simulink library "ros2lib"  (R2025a)
settings: Solver=ode45  StartTime=0.0  StopTime=10.0  RelTol=1e-3  EnableMultiTasking=on
undefined symbols (not defined in the file): coder, count, data, data_SL_Info, datatype, encoding, encoding_SL_Info, fields, fields_SL_Info, header, height, name, name_SL_Info, offset, point_step, ros, row_step, width
libraries: $bdroot x3
(part 1 of 2)
settings Model: Creator=The MathWorks, Inc.  LastModifiedBy=The MathWorks, Inc.
settings SolverCC: AlgebraicLoopSolver=TrustRegion  MaxZcPerStep=1.0
settings DataIOCC: LimitDataPoints=on  SaveFormat=Array  ReturnWorkspaceOutputs=off
settings OptimizationCC: ReuseModelBlockBuffer=off  LifeSpan=inf
settings DebuggingCC: SolverPrmCheckMsg=warning  UnconnectedInputMsg=warning  UnconnectedOutputMsg=warning  UnconnectedLineMsg=warning  AllowSymbolicDim=off  PregeneratedLibrarySubsystemCodeDiagnostic=none  SubsystemReferenceDiagnosticForUnitTest=warning  SFUnexpectedBacktrackingDiag=warning  SFNoUnconditionalDefaultTransitionDiag=warning  SFExecutionAtInitializationDiag=none  ArithmeticOperatorsInVariantConditions=warning
settings HardwareCC: ProdBitPerPointer=32.0  ProdBitPerSizeT=32.0  ProdBitPerPtrDiffT=32.0  ProdLargestAtomicFloat=None  ProdIntDivRoundTo=Undefined  ProdEndianess=Unspecified  ProdWordSize=32.0  ProdHWDeviceType=32-bit Generic
settings ModelReferenceCC: EnableRefExpFcnMdlSchedulingChecks=on  PropagateSignalLabelsOutOfModel=off
settings SFSimCC: SimUseLocalCustomCode=off
settings RTWCC: RTWUseLocalCustomCode=off  GPUComputeCapability=3.5  DLArmComputeVersion=19.05
settings CodeAppCC: StateflowObjectComments=on
settings GRTTargetCC: TargetLangStandard=C89/C90 (ANSI)
settings ConfigComp: CovScope=ReferencedModels  CovMetricSettings=dw  CovSaveCumulativeToWorkspaceVar=on  CovSaveSingleToWorkspaceVar=on  CovExternalEMLEnable=off  CovSFcnEnable=off

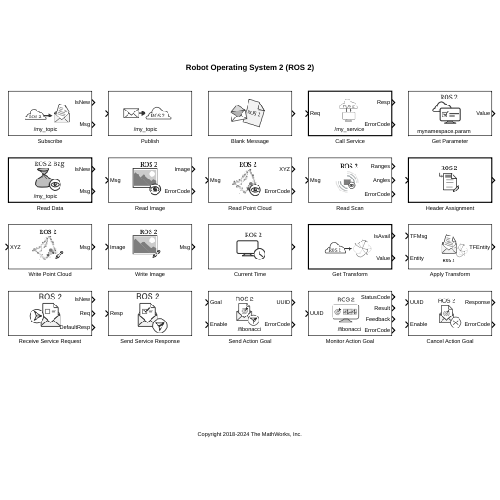
[thumbnail: Simulink's stored preview of the top-level diagram]
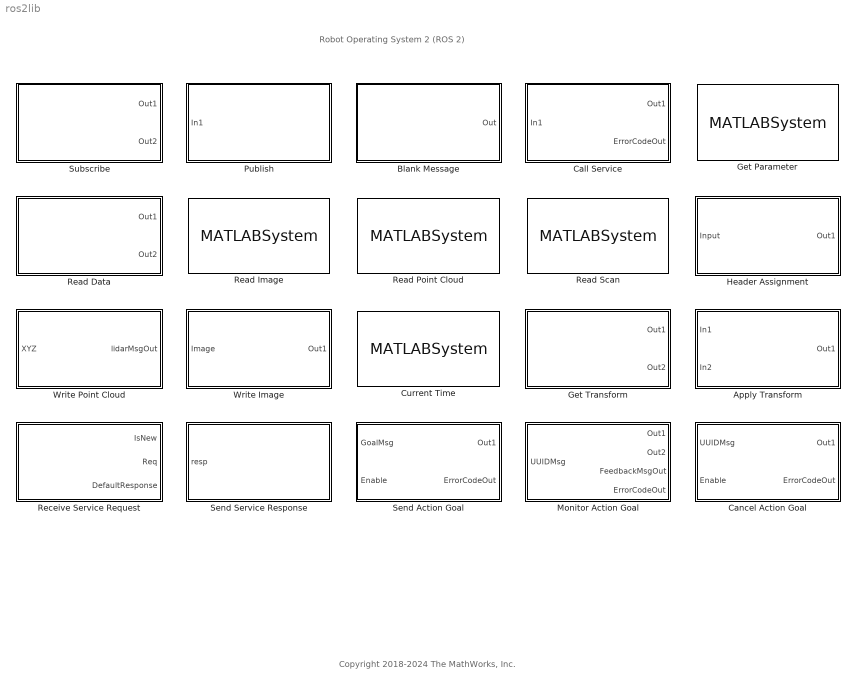
== system ros2lib ==
  note: Copyright 2018-2024 The MathWorks, Inc.
  note: Robot Operating System 2 (ROS 2)
  Apply Transform : Subsystem  InitFcn=ros.slros.internal.block.errorIfBlocksConflict(bdroot(gcb));  SystemSampleTime=SampleTime  mask(ros.slros2.internal.block.ApplyTransform){EntityMsgType=geometry_msgs/QuaternionStamped, SampleTime=-1}
      mask prompts: EntityMsgType "ros:slros2:blockmask:EntityMsgPrompt"; SampleTime "Simulink:blkprm_prompts:AllBlksSampleTime"
      mask help: ros:slros2:blockmask:ApplyTransformDescription
      mask init:
      | ros.slros2.internal.block.ApplyTransformBlockMask.dispatch('maskInitialize', gcb);
      settings: ModelCloseFcn=ros.slros2.internal.bus.Util.clearSLBusesInGlobalScope(gcb);
      mask Help: eval('ros.slros.internal.helpview(''ros2ApplyTransformBlock'')');
      mask TypeOptions EntityMsgType: ApplyTransform/EntityMsgType
      mask Callback EntityMsgType: ros.slros2.internal.block.ApplyTransformBlockMask.dispatch('entityMsgTypeSelect', gcb);
      mask TypeOptions SampleTime: SystemSampleTime
      mask DialogControl DescGroupVar Prompt: ros:slros2:blockmask:ApplyTransformMaskTitle
      mask DialogControl DescTextVar Prompt: ros:slros2:blockmask:ApplyTransformDescription
      mask DialogControl EntityMsgType Prompt: Entity message type:
      mask DialogControl SampleTime Prompt: Sample time (-1 for inherited):
      mask Display:
      | color('black');
      | port_label('input', 1, 'TFMsg');
      | port_label('input', 2, 'Entity');
      | port_label('output', 1, 'TFEntity');
  Blank Message : Subsystem  LoadFcn=ros.slros2.internal.block.MessageBlockMask.messageLoadFcn(gcb);  InitFcn=ros.slros.internal.block.errorIfBlocksConflict(bdroot(gcb));  mask(ROS2 Blank Message){messageClass=Message, entityType=geometry_msgs/Point, messageType=geometry_msgs/Point, SampleTime=inf}
      mask prompts: messageClass "ros:slros:blockmask:MessageClassPrompt"; entityType "ros:slros:blockmask:TypePrompt"; messageType "ros:slros:blockmask:FullTypePrompt"; SampleTime "Simulink:blkprm_prompts:AllSrcBlksSampleTime"
      mask help: ros:slros2:blockmask:BlankMsgDescription
      mask init:
      | ros.slros2.internal.block.MessageBlockMask.dispatch('maskInitialize', gcb);
      settings: ModelCloseFcn=ros.slros2.internal.bus.Util.clearSLBusesInGlobalScope(gcb);
      mask Help: eval('ros.slros.internal.helpview(''ros2BlankMsgBlock'')');
      mask TypeOptions messageClass: ros:slros:blockmask:MessageType_Msg | ros:slros:blockmask:MessageType_SrvReq | ros:slros:blockmask:MessageType_SrvResp | ros:slros:blockmask:MessageType_ActFb | ros:slros:blockmask:MessageType_ActGoal | ros:slros:blockmask:MessageType_ActRes
      mask Callback messageClass: ros.slros2.internal.block.MessageBlockMask.dispatch('messageClassChange', gcb);
      mask Callback entityType: ros.slros2.internal.block.MessageBlockMask.dispatch('entityTypeEdit', gcb);
      mask TypeOptions SampleTime: Constant/SampleTime
      mask DialogControl messageClass Prompt: Class:
      mask DialogControl entityType Prompt: Type:
      mask DialogControl id_msgTypeSelectBtn Prompt: ros:slros:blockmask:SelectPrompt
      mask DialogControl id_msgTypeSelectBtn Callback: ros.slros2.internal.block.MessageBlockMask.dispatch('selectButtonPressed', gcb);
      mask DialogControl messageType Prompt: Fully resolved type:
      mask DialogControl SampleTime Prompt: Sample time:
      mask Display: color('black');
  Call Service : Subsystem  LoadFcn=ros.slros2.internal.block.ServiceCallBlockMask.messageLoadFcn(gcb);  InitFcn=ros.slros.internal.block.errorIfBlocksConflict(bdroot(gcb));  TreatAsAtomicUnit=on  mask(ROS2 Call Service){topicSource=Select from ROS network, service=/my_service, serviceType=std_srvs/Empty, connectionTimeout=5, ShowErrorCodeOutput=on, legacyBusStruct=off, QOSHistory=Keep last, QOSDepth=1, QOSReliability=Reliable, QOSDurability=Volatile, QOSDeadline=Inf, QOSLifespan=Inf, QOSLiveliness=Automatic, QOSLeaseDuration=Inf, QOSAvoidROSNamespaceConventions=off}
      mask prompts: topicSource "ros:slros:svccaller:SourcePrompt"; service "ros:slros:svccaller:NamePrompt"; serviceType "ros:slros:svccaller:TypePrompt"; connectionTimeout "ros:slros:svccaller:ConnectionTimeoutPrompt"; ShowErrorCodeOutput "ros:slros:blockmask:ShowErrorCodePrompt"; legacyBusStruct "Use legacy bus structure"; QOSHistory "ros:slros2:blockmask:QOSHistoryPrompt"; QOSDepth "ros:slros2:blockmask:QOSDepthPrompt"; QOSReliability "ros:slros2:blockmask:QOSReliabilityPrompt"; QOSDurability "ros:slros2:blockmask:QOSDurabilityPrompt"; QOSDeadline "ros:slros2:blockmask:QOSDeadlinePrompt"; QOSLifespan "ros:slros2:blockmask:QOSLifespanPrompt"; QOSLiveliness "ros:slros2:blockmask:QOSLivelinessPrompt"; QOSLeaseDuration "ros:slros2:blockmask:QOSLeaseDurationPrompt"; QOSAvoidROSNamespaceConventions "ros:slros2:blockmask:QOSAvoidROSNamespaceConventionsPrompt"
      mask help: ros:slros2:blockmask:ServiceCallerDescription
      mask init:
      | ros.slros2.internal.block.ServiceCallBlockMask.dispatch('maskInitialize', gcb);
      settings: ModelCloseFcn=ros.slros2.internal.bus.Util.clearSLBusesInGlobalScope(gcb);
      mask Help: eval('ros.slros.internal.helpview(''ros2CallServiceBlock'')');
      mask TypeOptions topicSource: ros:slros:blockmask:TopicSourceFromNetwork | ros:slros:blockmask:TopicSourceSpecifyOwn
      mask Callback topicSource: ros.slros2.internal.block.ServiceCallBlockMask.dispatch('serviceSourceSelect', gcb);
      mask Callback service: ros.slros2.internal.block.ServiceCallBlockMask.dispatch('serviceEdit', gcb);
      mask Callback connectionTimeout: ros.slros2.internal.block.ServiceCallBlockMask.dispatch('connectionTimeoutEdit', gcb);
      mask TypeOptions QOSHistory: ServiceCaller/QOSHistory
      mask Callback QOSHistory: ros.slros2.internal.block.QOSSettingsMask.qosHistorySelect(gcb);
      mask TypeOptions QOSDepth: ServiceCaller/QOSDepth
      mask TypeOptions QOSReliability: ServiceCaller/QOSReliability
      mask TypeOptions QOSDurability: ServiceCaller/QOSDurability
      mask TypeOptions QOSDeadline: ServiceCaller/QOSDeadline
      mask TypeOptions QOSLifespan: ServiceCaller/QOSLifespan
      mask TypeOptions QOSLiveliness: ServiceCaller/QOSLiveliness
      mask TypeOptions QOSLeaseDuration: ServiceCaller/QOSLeaseDuration
      mask TypeOptions QOSAvoidROSNamespaceConventions: ServiceCaller/QOSAvoidROSNamespaceConventions
      mask DialogControl id_netAddrLink Prompt: ros:slros2:blockmask:ConfigNetworkAddrLinkText
      mask DialogControl id_netAddrLink Callback: ros.slros2.internal.block.SubscribeBlockMask.dispatch('configureNetworkAddrDlg', gcb);
      mask DialogControl Container6 Prompt: ros:slros2:blockmask:PubSubMainTab
      mask DialogControl topicSource Prompt: Source:
      mask DialogControl service Prompt: Name:
      mask DialogControl id_topicSelectBtn Prompt: ros:slros:blockmask:SelectPrompt
      mask DialogControl id_topicSelectBtn Callback: ros.slros2.internal.block.ServiceCallBlockMask.dispatch('serviceSelect', gcb, 'ros.slros2.internal.dlg.ServiceSelector');
      mask DialogControl serviceType Prompt: Type:
      mask DialogControl id_msgTypeSelectBtn Prompt: ros:slros:blockmask:SelectPrompt
      mask DialogControl id_msgTypeSelectBtn Callback: ros.slros2.internal.block.ServiceCallBlockMask.dispatch('serviceTypeSelect', gcb, 'ros.slros2.internal.dlg.ServiceTypeSelector');
      mask DialogControl connectionTimeout Prompt: Connection timeout:
      mask DialogControl ShowErrorCodeOutput Prompt: Show ErrorCode output port
      mask DialogControl id_cgContainer Prompt: ros:slros2:blockmask:PubSubQOSTab
      mask DialogControl QOSHistory Prompt: History:
      mask DialogControl QOSDepth Prompt: Depth:
      mask DialogControl QOSReliability Prompt: Reliability:
      mask DialogControl QOSDurability Prompt: Durability:
      mask DialogControl QOSDeadline Prompt: Deadline:
      mask DialogControl QOSLifespan Prompt: Lifespan:
      mask DialogControl QOSLiveliness Prompt: Liveliness:
      mask DialogControl QOSLeaseDuration Prompt: Lease Duration:
      mask DialogControl QOSAvoidROSNamespaceConventions Prompt: Avoid ROS Namespace Conventions
      mask Display:
      | color('black');
      | text(0.5, 0.15, '/my_service', 'horizontalAlignment', 'center');
      | port_label('input', 1, 'Req');
      | port_label('output', 1, 'Resp');
      | port_label('output', 2, 'ErrorCode');
  Cancel Action Goal : Subsystem  InitFcn=ros.slros.internal.ROSUtil.checkSendGoalBlkAvailability(gcb);  mask(ROS 2 Cancel Action Goal){ShowErrorCodeOutput=on, BlockId=ActCancel_ros2lib_244}
      mask prompts: ShowErrorCodeOutput "ros:slros2:blockmask:ShowErrorCodePortPrompt"; BlockId "Simulink Block Identifier:"
      mask help: ros:slros2:blockmask:CancelActionGoalDescription
      mask init:
      | ros.slros2.internal.block.CancelActionGoalBlockMask.dispatch('maskInitialize', gcb);
      settings: ModelCloseFcn=ros.slros2.internal.bus.Util.clearSLBusesInGlobalScope(gcb);
      mask Help: eval('ros.slros.internal.helpview("ros2CancelActionGoalBlock")')
      mask TypeOptions BlockId: CancelGoal/BlockId
      mask DialogControl ShowErrorCodeOutput Prompt: Show ErrorCode output port
      mask Display:
      | color('black');
      | port_label('input', 1, 'UUID');
      | port_label('input', 2, 'Enable');
      | port_label('output', 1, 'Response');
      | port_label('output', 2, 'ErrorCode');
  Current Time : MATLABSystem  InitFcn=ros.slros2.internal.block.CurrentTimeBlockMask.dispatch('initFcn', gcb);  System=ros.slros2.internal.block.CurrentTime  OutputFormat=bus  SampleTime=SampleTime  ModelName=untitled  mask(ros.slros2.internal.block.CurrentTime){OutputFormat=bus, SampleTime=-1, ModelName=untitled}
      mask prompts: OutputFormat "ros:slros:rostime:OutputFormatPrompt"; SampleTime "ros:slros:blockmask:SampleTimePrompt"; ModelName "ros:slros:blockmask:ModelNamePrompt"
      mask help: ros:slros2:blockmask:CurrentTimeMaskDescription
      settings: ModelCloseFcn=ros.slros2.internal.block.CurrentTimeBlockMask.dispatch('modelCloseFcn');
      mask Help: eval('ros.slros.internal.helpview(''ros2CurrentTimeBlock'')');
      mask TypeOptions OutputFormat: OutputFormat
      mask Callback OutputFormat: ros.slros2.internal.block.CurrentTimeBlockMask.dispatch('outputFormatSelect',gcb);
      mask TypeOptions SampleTime: SampleTime
      mask TypeOptions ModelName: ModelName
      mask DialogControl DescGroupVar Prompt: ros:slros2:blockmask:CurrentTimeMaskTitle
      mask DialogControl OutputFormat Prompt: Output format:
      mask DialogControl SampleTime Prompt: Sample time:
      mask DialogControl ModelName Prompt: Model name:
      mask Display: color('black')
  Get Parameter : MATLABSystem  System=ros.slros2.internal.block.GetParameter  ParameterName=mynamespace.param  ParameterType=double  ParameterMaxArrayLength=ParameterMaxArrayLength  ParameterInitialValue=ParameterInitialValue  SampleTime=SampleTime  ModelName=ros2lib  BlockId=ParamGet_ros2lib_196  mask(ros.slros2.internal.block.GetParameter){ParameterName=mynamespace.param, ParameterType=double, ParameterMaxArrayLength=16, ParameterInitialValue=0.0, SampleTime=-1, ModelName=ros2lib, BlockId=ParamGet_ros2lib_196}
      mask prompts: ParameterName "ros:slros:blockmask:ParameterNamePrompt"; ParameterType "ros:slros:blockmask:ParameterDataTypePrompt"; ParameterMaxArrayLength "ros:slros2:blockmask:GetParamMaxLenPrompt"; ParameterInitialValue "ros:slros:blockmask:ParameterInitialValuePrompt"; SampleTime "ros:slros:blockmask:SampleTimePrompt"; ModelName "Name of Simulink model:"; BlockId "Simulink Block Identifier:"
      mask help: ros:slros2:blockmask:GetParamMaskDescription
      mask Help: eval('ros.slros.internal.helpview(''ros2GetParameterBlock'')');
      mask TypeOptions ParameterName: ParameterName
      mask TypeOptions ParameterType: ParameterType
      mask Callback ParameterType: ros.slros2.internal.block.GetParameterBlockMask.dispatch('setParameterType',gcb);
      mask TypeOptions ParameterMaxArrayLength: ParameterMaxArrayLength
      mask TypeOptions ParameterInitialValue: ParameterInitialValue
      mask TypeOptions SampleTime: SampleTime
      mask TypeOptions ModelName: ModelName
      mask TypeOptions BlockId: BlockId
      mask DialogControl DescGroupVar Prompt: ros:slros2:blockmask:GetParamMaskTitle
      mask DialogControl id_netAddrLink Prompt: ros:slros2:blockmask:ConfigNetworkAddrLinkText
      mask DialogControl id_netAddrLink Callback: ros.slros2.internal.block.SubscribeBlockMask.dispatch('configureNetworkAddrDlg', gcb);
      mask DialogControl ROS2ParameterContainer Prompt: ros:slros2:blockmask:ParamContainerTitle
      mask DialogControl ParameterName Prompt: Name:
      mask DialogControl ParameterType Prompt: Data type:
      mask DialogControl ParameterMaxArrayLength Prompt: Maximum length:
      mask DialogControl ParameterInitialValue Prompt: Initial value:
      mask DialogControl SampleTime Prompt: Sample time:
  Get Transform : Subsystem  InitFcn=ros.slros.internal.block.errorIfBlocksConflict(bdroot(gcb));  TreatAsAtomicUnit=on  mask(ros.slros2.internal.block.GetTransform){FrameSource=Select from ROS network, TargetFrame=, SourceFrame=, OutputFormat=bus, SampleTime=-1, DynamicQoSHistory=Keep last, DynamicQoSDepth=1, DynamicQoSReliability=Reliable, DynamicQoSDurability=Volatile, DynamicQoSDeadline=Inf, DynamicQoSLifespan=Inf, DynamicQoSLiveliness=Automatic, DynamicQoSLeaseDuration=Inf, DynamicQoSAvoidROSNamespaceConventions=off, StaticQoSHistory=Keep last, StaticQoSDepth=1, StaticQoSReliability=Reliable, StaticQoSDurability=Volatile, StaticQoSDeadline=Inf, StaticQoSLifespan=Inf, StaticQoSLiveliness=Automatic, StaticQoSLeaseDuration=Inf, StaticQoSAvoidROSNamespaceConventions=off}
      mask prompts: FrameSource "ros:slros2:blockmask:FrameSourcePrompt"; TargetFrame "ros:slros2:blockmask:TargetPrompt"; SourceFrame "ros:slros2:blockmask:SourcePrompt"; OutputFormat "ros:slros2:blockmask:OutputFormatPrompt"; SampleTime "Simulink:blkprm_prompts:AllSrcBlksSampleTime"; DynamicQoSHistory "ros:slros2:blockmask:QOSHistoryPrompt"; DynamicQoSDepth "ros:slros2:blockmask:QOSDepthPrompt"; DynamicQoSReliability "ros:slros2:blockmask:QOSReliabilityPrompt"; DynamicQoSDurability "ros:slros2:blockmask:QOSDurabilityPrompt"; DynamicQoSDeadline "ros:slros2:blockmask:QOSDeadlinePrompt"; DynamicQoSLifespan "ros:slros2:blockmask:QOSLifespanPrompt"; DynamicQoSLiveliness "ros:slros2:blockmask:QOSLivelinessPrompt"; DynamicQoSLeaseDuration "ros:slros2:blockmask:QOSLeaseDurationPrompt"; DynamicQoSAvoidROSNamespaceConventions "ros:slros2:blockmask:QOSAvoidROSNamespaceConventionsPrompt"; StaticQoSHistory "ros:slros2:blockmask:QOSHistoryPrompt"; StaticQoSDepth "ros:slros2:blockmask:QOSDepthPrompt"; StaticQoSReliability "ros:slros2:blockmask:QOSReliabilityPrompt"; StaticQoSDurability "ros:slros2:blockmask:QOSDurabilityPrompt"; StaticQoSDeadline "ros:slros2:blockmask:QOSDeadlinePrompt"; StaticQoSLifespan "ros:slros2:blockmask:QOSLifespanPrompt"; StaticQoSLiveliness "ros:slros2:blockmask:QOSLivelinessPrompt"; StaticQoSLeaseDuration "ros:slros2:blockmask:QOSLeaseDurationPrompt"; StaticQoSAvoidROSNamespaceConventions "ros:slros2:blockmask:QOSAvoidROSNamespaceConventionsPrompt"
      mask help: ros:slros2:blockmask:GetTransformDescription
      mask init:
      | ros.slros2.internal.block.GetTransformBlockMask.dispatch('maskInitialize',gcb);
      settings: ModelCloseFcn=ros.slros2.internal.bus.Util.clearSLBusesInGlobalScope(gcb);
      mask Help: eval('ros.slros.internal.helpview(''ros2GetTransformBlock'')');
      mask TypeOptions FrameSource: ros:slros:blockmask:TopicSourceFromNetwork | ros:slros:blockmask:TopicSourceSpecifyOwn
      mask Callback FrameSource: ros.slros2.internal.block.GetTransformBlockMask.dispatch('frameSourceSelect',gcb);
      mask TypeOptions TargetFrame: SourceBlock/TargetFrame
      mask TypeOptions SourceFrame: SourceBlock/SourceFrame
      mask TypeOptions OutputFormat: SourceBlock/OutputFormat
      mask TypeOptions SampleTime: Constant/SampleTime
      mask TypeOptions DynamicQoSHistory: SourceBlock/DynamicQoSHistory
      mask Callback DynamicQoSHistory: ros.slros2.internal.block.GetTransformBlockMask.dispatch('qosHistorySelect',gcb,'Dynamic');
      mask TypeOptions DynamicQoSDepth: SourceBlock/DynamicQoSDepth
      mask TypeOptions DynamicQoSReliability: SourceBlock/DynamicQoSReliability
      mask TypeOptions DynamicQoSDurability: SourceBlock/DynamicQoSDurability
      mask TypeOptions DynamicQoSDeadline: SourceBlock/DynamicQOSDeadline
      mask TypeOptions DynamicQoSLifespan: SourceBlock/DynamicQOSLifespan
      mask TypeOptions DynamicQoSLiveliness: SourceBlock/DynamicQOSLiveliness
      mask TypeOptions DynamicQoSLeaseDuration: SourceBlock/DynamicQOSLeaseDuration
      mask TypeOptions DynamicQoSAvoidROSNamespaceConventions: SourceBlock/DynamicQOSAvoidROSNamespaceConventions
      mask TypeOptions StaticQoSHistory: SourceBlock/StaticQoSHistory
      mask Callback StaticQoSHistory: ros.slros2.internal.block.GetTransformBlockMask.dispatch('qosHistorySelect',gcb,'Static');
      mask TypeOptions StaticQoSDepth: SourceBlock/StaticQoSDepth
      mask TypeOptions StaticQoSReliability: SourceBlock/StaticQoSReliability
      mask TypeOptions StaticQoSDurability: SourceBlock/StaticQoSDurability
      mask TypeOptions StaticQoSDeadline: SourceBlock/StaticQOSDeadline
      mask TypeOptions StaticQoSLifespan: SourceBlock/StaticQOSLifespan
      mask TypeOptions StaticQoSLiveliness: SourceBlock/StaticQOSLiveliness
      mask TypeOptions StaticQoSLeaseDuration: SourceBlock/StaticQOSLeaseDuration
      mask TypeOptions StaticQoSAvoidROSNamespaceConventions: SourceBlock/StaticQOSAvoidROSNamespaceConventions
      mask DialogControl DescGroupVar Prompt: ros:slros2:blockmask:GetTransformMaskTitle
      mask DialogControl Container4 Prompt: ros:slros2:blockmask:PubSubMainTab
      mask DialogControl FrameSource Prompt: Frame source:
      mask DialogControl TargetFrame Prompt: Target:
      mask DialogControl id_targetSelectBtn Prompt: ros:slros2:blockmask:SelectPrompt
      mask DialogControl id_targetSelectBtn Callback: ros.slros2.internal.block.GetTransformBlockMask.dispatch('frameSelect',gcb,'TargetFrame','ros.slros2.internal.dlg.FrameSelector');
      mask DialogControl SourceFrame Prompt: Source:
      mask DialogControl id_sourceSelectBtn Prompt: ros:slros2:blockmask:SelectPrompt
      mask DialogControl id_sourceSelectBtn Callback: ros.slros2.internal.block.GetTransformBlockMask.dispatch('frameSelect',gcb,'SourceFrame','ros.slros2.internal.dlg.FrameSelector');
      mask DialogControl OutputFormat Prompt: Output format:
      mask DialogControl SampleTime Prompt: Sample time:
      mask DialogControl Container5 Prompt: ros:slros2:blockmask:PubSubQOSTab
      mask DialogControl Container6 Prompt: ros:slros2:blockmask:DynamicListenerQoSPrompt
      mask DialogControl DynamicQoSHistory Prompt: History:
      mask DialogControl DynamicQoSDepth Prompt: Depth:
      mask DialogControl DynamicQoSReliability Prompt: Reliability:
      mask DialogControl DynamicQoSDurability Prompt: Durability:
      mask DialogControl DynamicQoSDeadline Prompt: Deadline:
      mask DialogControl DynamicQoSLifespan Prompt: Lifespan:
      mask DialogControl DynamicQoSLiveliness Prompt: Liveliness:
      mask DialogControl DynamicQoSLeaseDuration Prompt: Lease Duration:
      mask DialogControl DynamicQoSAvoidROSNamespaceConventions Prompt: Avoid ROS Namespace Conventions
      mask DialogControl Container7 Prompt: ros:slros2:blockmask:StaticListenerQoSPrompt
      mask DialogControl StaticQoSHistory Prompt: History:
      mask DialogControl StaticQoSDepth Prompt: Depth:
      mask DialogControl StaticQoSReliability Prompt: Reliability:
      mask DialogControl StaticQoSDurability Prompt: Durability:
      mask DialogControl StaticQoSDeadline Prompt: Deadline:
      mask DialogControl StaticQoSLifespan Prompt: Lifespan:
      mask DialogControl StaticQoSLiveliness Prompt: Liveliness:
      mask DialogControl StaticQoSLeaseDuration Prompt: Lease Duration:
      mask DialogControl StaticQoSAvoidROSNamespaceConventions Prompt: Avoid ROS Namespace Conventions
      mask Display:
      | color('black');
      | port_label('output', 1, 'IsAvail');
      | port_label('output', 2, 'Value');
  Header Assignment : Subsystem  TreatAsAtomicUnit=on  mask(ROS2 Header){SetFrameID=off, FrameID=, InsertTimeStamp=off, SetHeaderFieldName=Use the default header field name, HeaderFieldName=header}
      mask prompts: SetFrameID "ros:slros2:blockmask:SetFrameIdPrompt"; InsertTimeStamp "ros:slros2:blockmask:SetTimestampPrompt"; SetHeaderFieldName "ros:slros2:blockmask:SetHdrFldNamePrompt"
      mask help: ros:slros2:blockmask:HdrAssignDescription
      mask init:
      | ros.slros2.internal.block.HeaderAssignmentBlockMask.dispatch('maskInitialize',gcb);
      mask Help: eval('ros.slros.internal.helpview("ros2HeaderAssignment")');
      mask Callback SetFrameID: ros.slros2.internal.block.HeaderAssignmentBlockMask.dispatch('checkSetFrameId',gcb);
      mask Callback FrameID: ros.slros2.internal.block.HeaderAssignmentBlockMask.dispatch('setFrameId',gcb);
      mask TypeOptions SetHeaderFieldName: ros:slros2:blockmask:HdrFldNameDefault | ros:slros2:blockmask:HdrFldNameSpecifyOwn
      mask Callback SetHeaderFieldName: ros.slros2.internal.block.HeaderAssignmentBlockMask.dispatch('checkSetHeaderFieldName',gcb);
      mask Callback HeaderFieldName: ros.slros2.internal.block.HeaderAssignmentBlockMask.dispatch('setHeaderFieldName',gcb);
      mask DialogControl SetFrameID Prompt: Set Frame ID:
      mask DialogControl InsertTimeStamp Prompt: Set Timestamp
      mask DialogControl SetHeaderFieldName Prompt: Header field name:
      mask Display:
      | color('white');
      | 
      | plot([100,100,100,100],[100,100,100,100]);
      | 
      | plot([0,0,0,0],[0,0,0,0]);
  Monitor Action Goal : Subsystem  LoadFcn=ros.slros2.internal.bus.Util.clearSLBusesInGlobalScope(gcb);  InitFcn=|  mask(ROS 2 Monitor Action Goal){action=/fibonacci, actionType=example_interfaces/Fibonacci, ShowFeedbackOutput=on, ShowErrorCodeOutput=on, BlockId=ActSend_ros2lib_226}
      | ros.slros.internal.block.errorIfBlocksConflict(bdroot(gcb));
      | ros.slros.internal.ROSUtil.checkSendGoalBlkPairAvailability(gcb);
      mask prompts: action "ros:slros2:blockmask:ActionNamePrompt"; actionType "ros:slros2:blockmask:ActionTypePrompt"; ShowFeedbackOutput "ros:slros2:blockmask:ShowFeedbackPortPrompt"; ShowErrorCodeOutput "ros:slros2:blockmask:ShowErrorCodePortPrompt"; BlockId "Simulink Block Identifier:"
      mask help: ros:slros2:blockmask:MonitorActionGoalDescription
      mask init:
      | ros.slros2.internal.block.MonitorActionGoalBlockMask.dispatch('maskInitialize',gcb);
      settings: CopyFcn=ros.slros2.internal.block.MonitorActionGoalBlockMask.dispatch('copyBlockInit',gcb);  DeleteFcn=ros.slros.internal.ROSUtil.removeBlkPairingRegistration(gcb);
      mask Help: eval('ros.slros.internal.helpview("ros2MonitorActionGoalBlock")')
      mask TypeOptions action: MonitorGoal/ActionName
      mask Callback action: ros.slros2.internal.block.MonitorActionGoalBlockMask.dispatch('updateSubsystem',gcb);
      mask TypeOptions actionType: MonitorGoal/ActionType
      mask Callback actionType: ros.slros2.internal.block.MonitorActionGoalBlockMask.dispatch('updateSubsystem',gcb);
      mask TypeOptions BlockId: MonitorGoal/BlockId
      mask DialogControl action Prompt: Name:
      mask DialogControl actionType Prompt: Type:
      mask DialogControl PairedBlkText Prompt: ros:slros2:blockmask:PairedSendGoalBlkPrompt
      mask DialogControl PairedBlkLink Prompt: ros2lib/Send Action Goal
      mask DialogControl PairedBlkLink Callback: ros.slros.internal.ROSUtil.addMonitorAndSendActionGoalBlockPair(bdroot,'ros2lib/Send Action Goal',gcb);
      mask DialogControl ShowFeedbackOutput Prompt: Show Feedback output port
      mask DialogControl ShowErrorCodeOutput Prompt: Show ErrorCode output port
      mask Display:
      | color('black');
      | text(0.5, 0.15, '/fibonacci', 'horizontalAlignment', 'center');
      | port_label('input', 1, 'UUID');
      | port_label('output', 1, 'StatusCode');
      | port_label('output', 2, 'Result');
      | port_label('output', 3, 'Feedback');
      | port_label('output', 4, 'ErrorCode');
  Publish : Subsystem  LoadFcn=ros.slros2.internal.block.PublishBlockMask.messageLoadFcn(gcb);  InitFcn=ros.slros.internal.block.errorIfBlocksConflict(bdroot(gcb));  mask(ROS2 Publish){topicSource=Select from ROS network, topic=/my_topic, messageType=geometry_msgs/Point, QOSHistory=Keep last, QOSDepth=10, QOSReliability=Reliable, QOSDurability=Volatile, QOSDeadline=Inf, QOSLifespan=Inf, QOSLiveliness=Automatic, QOSLeaseDuration=Inf, QOSAvoidROSNamespaceConventions=off}
      mask prompts: topicSource "ros:slros:blockmask:TopicSourcePrompt"; topic "ros:slros:blockmask:TopicPrompt"; messageType "ros:slros:blockmask:MessageTypePrompt"; QOSHistory "ros:slros2:blockmask:QOSHistoryPrompt"; QOSDepth "ros:slros2:blockmask:QOSDepthPrompt"; QOSReliability "ros:slros2:blockmask:QOSReliabilityPrompt"; QOSDurability "ros:slros2:blockmask:QOSDurabilityPrompt"; QOSDeadline "ros:slros2:blockmask:QOSDeadlinePrompt"; QOSLifespan "ros:slros2:blockmask:QOSLifespanPrompt"; QOSLiveliness "ros:slros2:blockmask:QOSLivelinessPrompt"; QOSLeaseDuration "ros:slros2:blockmask:QOSLeaseDurationPrompt"; QOSAvoidROSNamespaceConventions "ros:slros2:blockmask:QOSAvoidROSNamespaceConventionsPrompt"
      mask help: ros:slros:blockmask:PublisherDescription
      mask init:
      | ros.slros2.internal.block.PublishBlockMask.dispatch('maskInitialize', gcb);
      settings: ModelCloseFcn=ros.slros2.internal.bus.Util.clearSLBusesInGlobalScope(gcb);
      mask Help: eval('ros.slros.internal.helpview(''ros2PublishBlock'')');
      mask TypeOptions topicSource: ros:slros2:blockmask:TopicSourceFromNetwork | ros:slros2:blockmask:TopicSourceSpecifyOwn
      mask Callback topicSource: ros.slros2.internal.block.PublishBlockMask.dispatch('topicSourceSelect', gcb);
      mask Callback topic: ros.slros2.internal.block.PublishBlockMask.dispatch('topicEdit', gcb);
      mask Callback messageType: ros.slros2.internal.block.PublishBlockMask.dispatch('messageTypeEdit', gcb);
      mask TypeOptions QOSHistory: SinkBlock/QOSHistory
      mask Callback QOSHistory: ros.slros2.internal.block.QOSSettingsMask.qosHistorySelect(gcb);
      mask TypeOptions QOSDepth: SinkBlock/QOSDepth
      mask TypeOptions QOSReliability: SinkBlock/QOSReliability
      mask TypeOptions QOSDurability: SinkBlock/QOSDurability
      mask TypeOptions QOSDeadline: SinkBlock/QOSDeadline
      mask TypeOptions QOSLifespan: SinkBlock/QOSLifespan
      mask TypeOptions QOSLiveliness: SinkBlock/QOSLiveliness
      mask TypeOptions QOSLeaseDuration: SinkBlock/QOSLeaseDuration
      mask TypeOptions QOSAvoidROSNamespaceConventions: SinkBlock/QOSAvoidROSNamespaceConventions
      mask DialogControl id_netAddrLink Prompt: ros:slros2:blockmask:ConfigNetworkAddrLinkText
      mask DialogControl id_netAddrLink Callback: ros.slros2.internal.block.PublishBlockMask.dispatch('configureNetworkAddrDlg', gcb);
      mask DialogControl Container13 Prompt: ros:slros2:blockmask:PubSubMainTab
      mask DialogControl topicSource Prompt: Topic source:
      mask DialogControl topic Prompt: Topic:
      mask DialogControl id_topicSelectBtn Prompt: ros:slros:blockmask:SelectPrompt
      mask DialogControl id_topicSelectBtn Callback: ros.slros2.internal.block.PublishBlockMask.dispatch('topicSelect', gcb, 'ros.slros2.internal.dlg.TopicSelector');
      mask DialogControl messageType Prompt: Message type:
      mask DialogControl id_msgTypeSelectBtn Prompt: ros:slros:blockmask:SelectPrompt
      mask DialogControl id_msgTypeSelectBtn Callback: ros.slros2.internal.block.PublishBlockMask.dispatch('messageTypeSelect', gcb, 'ros.slros2.internal.dlg.MessageTypeSelector');
      mask DialogControl id_cgContainer Prompt: ros:slros2:blockmask:PubSubQOSTab
      mask DialogControl QOSHistory Prompt: History:
      mask DialogControl QOSDepth Prompt: Depth:
      mask DialogControl QOSReliability Prompt: Reliability:
      mask DialogControl QOSDurability Prompt: Durability:
      mask DialogControl QOSDeadline Prompt: Deadline:
      mask DialogControl QOSLifespan Prompt: Lifespan:
      mask DialogControl QOSLiveliness Prompt: Liveliness:
      mask DialogControl QOSLeaseDuration Prompt: Lease Duration:
      mask DialogControl QOSAvoidROSNamespaceConventions Prompt: Avoid ROS Namespace Conventions
      mask Display:
      | color('black');
      | text(0.45, 0.15, '/my_topic', 'horizontalAlignment', 'center');
  Read Data : Subsystem  InitFcn=ros.slros.internal.block.errorIfBlocksConflict(bdroot(gcb));  TreatAsAtomicUnit=on  mask(Read Data from ROS2 Bag){topic=/my_topic, sampleTime=-1, logfileType=rosbag2, modelName=ros2lib, msgType=}
      mask prompts: topic "ros:slros:readlog:TopicPrompt"; sampleTime "ros:slros:blockmask:SampleTimePrompt"
      mask help: ros:slros:readlog:ReadDataDescription
      mask init:
      | ros.slros.internal.block.ReadDataBlockMask.blockInitFcn(gcb);
      settings: ModelCloseFcn=ros.slros.internal.block.ReadDataBlockMask.modelCloseFcn(gcb);
      mask Help: eval('ros.slros.internal.helpview(''ros2ReadDataBlock'')');
      mask TypeOptions topic: SourceBlock/Topic
      mask TypeOptions sampleTime: SourceBlock/SampleTime
      mask TypeOptions logfileType: SourceBlock/LogfileType
      mask TypeOptions modelName: SourceBlock/ModelName
      mask TypeOptions msgType: SourceBlock/MsgType
      mask DialogControl id_logDataLink Prompt: ros:slros:readlog:LoadDataPrompt
      mask DialogControl id_logDataLink Callback: ros.slros.internal.block.ReadDataBlockMask.loadLogfileLink(gcb)
      mask DialogControl topic Prompt: Topic:
      mask DialogControl id_topicSelectBtn Prompt: ros:slros:readlog:SelectPrompt
      mask DialogControl id_topicSelectBtn Callback: ros.slros.internal.block.ReadDataBlockMask.topicSelectButton(gcb)
      mask DialogControl sampleTime Prompt: Sample time:
      mask Display:
      | color('black');
      | text(0.45, 0.15, '/my_topic', 'horizontalAlignment', 'center');
      | port_label('output', 1, 'IsNew');
      | port_label('output', 2, 'Msg');
  Read Image : MATLABSystem  InitFcn=ros.slros.internal.block.errorIfBlocksConflict(bdroot(gcb));  System=ros.slros2.internal.block.ReadImage  MaximumImageSize=[ 2000, 2000 ]  ImageEncoding=rgb8  ShowAlphaOutput=off  ShowErrorCodeOutput=on  VariableSizeOutputs=off
      mask Type: ros.slros2.internal.block.ReadImage
  Read Point Cloud : MATLABSystem  InitFcn=ros.slros.internal.block.errorIfBlocksConflict(bdroot(gcb));  System=ros.slros2.internal.block.ReadPointCloud  MaximumPointCloudSize=[480, 640]  PreserveStructure=off  ShowRGBOutput=off  ShowIntensityOutput=off  ShowErrorCodeOutput=on  VariableSizeOutputs=off
      mask Type: ros.slros2.internal.block.ReadPointCloud
  Read Scan : MATLABSystem  InitFcn=ros.slros.internal.block.errorIfBlocksConflict(bdroot(gcb));  System=ros.slros2.internal.block.ReadScan  MaximumArrayLength=100  ShowAnglesOutput=on  ShowIntensityOutput=off  ShowErrorCodeOutput=on  VariableSizeOutputs=off
      mask Type: ros.slros2.internal.block.ReadScan
  Receive Service Request : Subsystem  LoadFcn=ros.slros2.internal.block.ReceiveRequestBlockMask.messageLoadFcn(gcb);  InitFcn=|  StopFcn=ros.slros2.internal.block.ReceiveRequestBlockMask.clearServer(gcb);  mask(ROS2 Receive Service Request){service=/my_service, serviceType=std_srvs/Empty, SampleTime=-1, ShowDefaultRespOutput=on, BlockId=ServRec_ros2lib_224, QOSHistory=Keep last, QOSDepth=1, QOSReliability=Reliable, QOSDurability=Volatile, QOSDeadline=Inf, QOSLifespan=Inf, QOSLiveliness=Automatic, QOSLeaseDuration=Inf, QOSAvoidROSNamespaceConventions=off}
      | ros.slros.internal.block.errorIfBlocksConflict(bdroot(gcb));
      | ros.slros.internal.ROSUtil.checkSvcServerBlkAvailability(gcb);
      | ros.slros2.internal.block.ReceiveRequestBlockMask.initializeServer(gcb);
      mask prompts: service "ros:slros:svccaller:NamePrompt"; serviceType "ros:slros:svccaller:TypePrompt"; SampleTime "ros:slros:blockmask:SampleTimePrompt"; ShowDefaultRespOutput "ros:slros2:blockmask:ShowRespOutportPrompt"; BlockId "Simulink Block Identifier:"; QOSHistory "ros:slros2:blockmask:QOSHistoryPrompt"; QOSDepth "ros:slros2:blockmask:QOSDepthPrompt"; QOSReliability "ros:slros2:blockmask:QOSReliabilityPrompt"; QOSDurability "ros:slros2:blockmask:QOSDurabilityPrompt"; QOSDeadline "ros:slros2:blockmask:QOSDeadlinePrompt"; QOSLifespan "ros:slros2:blockmask:QOSLifespanPrompt"; QOSLiveliness "ros:slros2:blockmask:QOSLivelinessPrompt"; QOSLeaseDuration "ros:slros2:blockmask:QOSLeaseDurationPrompt"; QOSAvoidROSNamespaceConventions "ros:slros2:blockmask:QOSAvoidROSNamespaceConventionsPrompt"
      mask help: ros:slros2:blockmask:ReceiveRequestDescription
      mask init:
      | ros.slros2.internal.block.ReceiveRequestBlockMask.dispatch('maskInitialize', gcb);
      settings: CopyFcn=ros.slros2.internal.block.ReceiveRequestBlockMask.dispatch('copyBlockInit',gcb);  DeleteFcn=ros.slros2.internal.block.ReceiveRequestBlockMask.dispatch('deleteFcnCallback',gcb);  ModelCloseFcn=ros.slros2.internal.bus.Util.clearSLBusesInGlobalScope(gcb);  PreSaveFcn=ros.slros2.internal.block.ReceiveRequestBlockMask.clearServer(gcb);
      mask Help: eval('ros.slros.internal.helpview("ros2ReceiveRequestBlock")');
      mask TypeOptions service: SvcReceiverObj/ServiceName
      mask Callback service: ros.slros2.internal.block.ReceiveRequestBlockMask.dispatch('serviceEdit', gcb);
      mask TypeOptions serviceType: SvcReceiverObj/ServiceType
      mask TypeOptions SampleTime: Blank Message/SampleTime | Blank Message1/SampleTime
      mask TypeOptions BlockId: SvcReceiverObj/BlockId
      mask TypeOptions QOSHistory: SvcReceiverObj/QOSHistory
      mask Callback QOSHistory: ros.slros2.internal.block.QOSSettingsMask.qosHistorySelect(gcb);
      mask TypeOptions QOSDepth: SvcReceiverObj/QOSDepth
      mask TypeOptions QOSReliability: SvcReceiverObj/QOSReliability
      mask TypeOptions QOSDurability: SvcReceiverObj/QOSDurability
      mask TypeOptions QOSDeadline: SvcReceiverObj/QOSDeadline
      mask TypeOptions QOSLifespan: SvcReceiverObj/QOSLifespan
      mask TypeOptions QOSLiveliness: SvcReceiverObj/QOSLiveliness
      mask TypeOptions QOSLeaseDuration: SvcReceiverObj/QOSLeaseDuration
      mask TypeOptions QOSAvoidROSNamespaceConventions: SvcReceiverObj/QOSAvoidROSNamespaceConventions
      mask DialogControl id_netAddrLink Prompt: Configure ROS 2 Domain ID and ROS Middleware (RMW)
      mask DialogControl id_netAddrLink Callback: ros.slros2.internal.block.SubscribeBlockMask.dispatch('configureNetworkAddrDlg', gcb);
      mask DialogControl Container4 Prompt: ros:slros2:blockmask:PubSubMainTab
      mask DialogControl service Prompt: Name:
      mask DialogControl serviceType Prompt: Type:
      mask DialogControl id_msgTypeSelectBtn Prompt: ros:slros:blockmask:SelectPrompt
      mask DialogControl id_msgTypeSelectBtn Callback: ros.slros2.internal.block.ReceiveRequestBlockMask.dispatch('serviceTypeSelect', gcb, 'ros.slros2.internal.dlg.ServiceTypeSelector');
      mask DialogControl PairedBlkText Prompt: ros:slros2:blockmask:PairedSendBlkPrompt
      mask DialogControl PairedBlkLink Prompt: ros2lib/Send Service Response
      mask DialogControl PairedBlkLink Callback: ros.slros.internal.ROSUtil.addServerResponseBlockPair(bdroot, 'ros2lib/Send Service Response', gcb);
      mask DialogControl SampleTime Prompt: Sample time:
      mask DialogControl ShowDefaultRespOutput Prompt: Show Default Response output port
      mask DialogControl id_cgContainer Prompt: ros:slros2:blockmask:PubSubQOSTab
      mask DialogControl QOSHistory Prompt: History:
      mask DialogControl QOSDepth Prompt: Depth:
      mask DialogControl QOSReliability Prompt: Reliability:
      mask DialogControl QOSDurability Prompt: Durability:
      mask DialogControl QOSDeadline Prompt: Deadline:
      mask DialogControl QOSLifespan Prompt: Lifespan:
      mask DialogControl QOSLiveliness Prompt: Liveliness:
      mask DialogControl QOSLeaseDuration Prompt: Lease Duration:
      mask DialogControl QOSAvoidROSNamespaceConventions Prompt: Avoid ROS Namespace Conventions
      mask Display:
      | color('black');
      | text(0.5, 0.15, '/my_service', 'horizontalAlignment', 'center');
      | port_label('output', 1, 'IsNew');
      | port_label('output', 2, 'Req');
      | port_label('output', 3, 'DefaultResp');
  Send Action Goal : Subsystem  LoadFcn=ros.slros2.internal.block.SendActionGoalBlockMask.messageLoadFcn(gcb);  InitFcn=ros.slros.internal.block.errorIfBlocksConflict(bdroot(gcb));  mask(ROS 2 Send Action Goal){actionSource=Select from ROS network, action=/fibonacci, actionType=example_interfaces/Fibonacci, ShowErrorCodeOutput=on, BlockId=ActSend_ros2lib_226, GoalServiceQoSHistory=Keep last, GoalServiceQoSDepth=1, GoalServiceQoSReliability=Reliable, GoalServiceQoSDurability=Volatile, GoalServiceQoSDeadline=Inf, GoalServiceQoSLifespan=Inf, GoalServiceQoSLiveliness=Automatic, GoalServiceQoSLeaseDuration=Inf, ResultServiceQoSHistory=Keep last, ResultServiceQoSDepth=1, ResultServiceQoSReliability=Reliable, ResultServiceQoSDurability=Volatile, ResultServiceQoSDeadline=Inf, ResultServiceQoSLifespan=Inf, ResultServiceQoSLiveliness=Automatic, ResultServiceQoSLeaseDuration=Inf, CancelServiceQoSHistory=Keep last, CancelServiceQoSDepth=1, CancelServiceQoSReliability=Reliable, CancelServiceQoSDurability=Volatile, CancelServiceQoSDeadline=Inf, CancelServiceQoSLifespan=Inf, CancelServiceQoSLiveliness=Automatic, CancelServiceQoSLeaseDuration=Inf, FeedbackTopicQoSHistory=Keep last, FeedbackTopicQoSReliability=Reliable, FeedbackTopicQoSDepth=1, FeedbackTopicQoSDurability=Volatile, FeedbackTopicQoSDeadline=Inf, FeedbackTopicQoSLifespan=Inf, FeedbackTopicQoSLiveliness=Automatic, FeedbackTopicQoSLeaseDuration=Inf, StatusTopicQoSHistory=Keep last, StatusTopicQoSDepth=1, StatusTopicQoSReliability=Reliable, StatusTopicQoSDurability=Transient local, StatusTopicQoSDeadline=Inf, StatusTopicQoSLifespan=Inf, StatusTopicQoSLiveliness=Automatic, StatusTopicQoSLeaseDuration=Inf}
      mask prompts: actionSource "ros:slros2:blockmask:ActionSourcePrompt"; action "ros:slros2:blockmask:ActionNamePrompt"; actionType "ros:slros2:blockmask:ActionTypePrompt"; ShowErrorCodeOutput "ros:slros2:blockmask:ShowErrorCodePortPrompt"; BlockId "Simulink Block Identifier:"; GoalServiceQoSHistory "ros:slros2:blockmask:QOSHistoryPrompt"; GoalServiceQoSDepth "ros:slros2:blockmask:QOSDepthPrompt"; GoalServiceQoSReliability "ros:slros2:blockmask:QOSReliabilityPrompt"; GoalServiceQoSDurability "ros:slros2:blockmask:QOSDurabilityPrompt"; GoalServiceQoSDeadline "ros:slros2:blockmask:QOSDeadlinePrompt"; GoalServiceQoSLifespan "ros:slros2:blockmask:QOSLifespanPrompt"; GoalServiceQoSLiveliness "ros:slros2:blockmask:QOSLivelinessPrompt"; GoalServiceQoSLeaseDuration "ros:slros2:blockmask:QOSLeaseDurationPrompt"; ResultServiceQoSHistory "ros:slros2:blockmask:QOSHistoryPrompt"; ResultServiceQoSDepth "ros:slros2:blockmask:QOSDepthPrompt"; ResultServiceQoSReliability "ros:slros2:blockmask:QOSReliabilityPrompt"; ResultServiceQoSDurability "ros:slros2:blockmask:QOSDurabilityPrompt"; ResultServiceQoSDeadline "ros:slros2:blockmask:QOSDeadlinePrompt"; ResultServiceQoSLifespan "ros:slros2:blockmask:QOSLifespanPrompt"; ResultServiceQoSLiveliness "ros:slros2:blockmask:QOSLivelinessPrompt"; ResultServiceQoSLeaseDuration "ros:slros2:blockmask:QOSLeaseDurationPrompt"; CancelServiceQoSHistory "ros:slros2:blockmask:QOSHistoryPrompt"; CancelServiceQoSDepth "ros:slros2:blockmask:QOSDepthPrompt"; CancelServiceQoSReliability "ros:slros2:blockmask:QOSReliabilityPrompt"; CancelServiceQoSDurability "ros:slros2:blockmask:QOSDurabilityPrompt"; CancelServiceQoSDeadline "ros:slros2:blockmask:QOSDeadlinePrompt"; CancelServiceQoSLifespan "ros:slros2:blockmask:QOSLifespanPrompt"; CancelServiceQoSLiveliness "ros:slros2:blockmask:QOSLivelinessPrompt"; CancelServiceQoSLeaseDuration "ros:slros2:blockmask:QOSLeaseDurationPrompt"; FeedbackTopicQoSHistory "ros:slros2:blockmask:QOSHistoryPrompt"; FeedbackTopicQoSReliability "ros:slros2:blockmask:QOSReliabilityPrompt"; FeedbackTopicQoSDepth "ros:slros2:blockmask:QOSDepthPrompt"; FeedbackTopicQoSDurability "ros:slros2:blockmask:QOSDurabilityPrompt"; FeedbackTopicQoSDeadline "ros:slros2:blockmask:QOSDeadlinePrompt"; FeedbackTopicQoSLifespan "ros:slros2:blockmask:QOSLifespanPrompt"; FeedbackTopicQoSLiveliness "ros:slros2:blockmask:QOSLivelinessPrompt"; FeedbackTopicQoSLeaseDuration "ros:slros2:blockmask:QOSLeaseDurationPrompt"; StatusTopicQoSHistory "ros:slros2:blockmask:QOSHistoryPrompt"; StatusTopicQoSDepth "ros:slros2:blockmask:QOSDepthPrompt"; StatusTopicQoSReliability "ros:slros2:blockmask:QOSReliabilityPrompt"; StatusTopicQoSDurability "ros:slros2:blockmask:QOSDurabilityPrompt"; StatusTopicQoSDeadline "ros:slros2:blockmask:QOSDeadlinePrompt"; StatusTopicQoSLifespan "ros:slros2:blockmask:QOSLifespanPrompt"; StatusTopicQoSLiveliness "ros:slros2:blockmask:QOSLivelinessPrompt"; StatusTopicQoSLeaseDuration "ros:slros2:blockmask:QOSLeaseDurationPrompt"
      mask help: ros:slros2:blockmask:SendActionGoalDescription
      mask init:
      | ros.slros2.internal.block.SendActionGoalBlockMask.dispatch('maskInitialize',gcb);
      settings: CopyFcn=ros.slros2.internal.block.SendActionGoalBlockMask.dispatch('copyBlockInit',gcb);  DeleteFcn=ros.slros.internal.ROSUtil.removeBlkPairingRegistration(gcb);  ModelCloseFcn=ros.slros2.internal.bus.Util.clearSLBusesInGlobalScope(gcb);
      mask Help: eval('ros.slros.internal.helpview("ros2SendActionGoalBlock")');
      mask TypeOptions actionSource: ros:slros:blockmask:TopicSourceFromNetwork | ros:slros:blockmask:TopicSourceSpecifyOwn
      mask Callback actionSource: ros.slros2.internal.block.SendActionGoalBlockMask.dispatch('actionSourceSelect',gcb);
      mask Callback action: ros.slros2.internal.block.SendActionGoalBlockMask.dispatch('actionEdit',gcb);
      mask TypeOptions BlockId: SendGoal/BlockId
      mask TypeOptions GoalServiceQoSHistory: SendGoal/GoalServiceQoSHistory
      mask Callback GoalServiceQoSHistory: ros.slros2.internal.block.SendActionGoalBlockMask.dispatch('qosHistorySelect',gcb,'GoalService');
      mask TypeOptions GoalServiceQoSDepth: SendGoal/GoalServiceQoSDepth
      mask TypeOptions GoalServiceQoSReliability: SendGoal/GoalServiceQoSReliability
      mask TypeOptions GoalServiceQoSDurability: SendGoal/GoalServiceQoSDurability
      mask TypeOptions GoalServiceQoSDeadline: SendGoal/GoalServiceQoSDeadline
      mask TypeOptions GoalServiceQoSLifespan: SendGoal/GoalServiceQoSLifespan
      mask TypeOptions GoalServiceQoSLiveliness: SendGoal/GoalServiceQoSLiveliness
      mask TypeOptions GoalServiceQoSLeaseDuration: SendGoal/GoalServiceQoSLeaseDuration
      mask TypeOptions ResultServiceQoSHistory: SendGoal/ResultServiceQoSHistory
      mask Callback ResultServiceQoSHistory: ros.slros2.internal.block.SendActionGoalBlockMask.dispatch('qosHistorySelect',gcb,'ResultService');
      mask TypeOptions ResultServiceQoSDepth: SendGoal/ResultServiceQoSDepth
      mask TypeOptions ResultServiceQoSReliability: SendGoal/ResultServiceQoSReliability
      mask TypeOptions ResultServiceQoSDurability: SendGoal/ResultServiceQoSDurability
      mask TypeOptions ResultServiceQoSDeadline: SendGoal/ResultServiceQoSDeadline
      mask TypeOptions ResultServiceQoSLifespan: SendGoal/ResultServiceQoSLifespan
      mask TypeOptions ResultServiceQoSLiveliness: SendGoal/ResultServiceQoSLiveliness
      mask TypeOptions ResultServiceQoSLeaseDuration: SendGoal/ResultServiceQoSLeaseDuration
      mask TypeOptions CancelServiceQoSHistory: SendGoal/CancelServiceQoSHistory
      mask Callback CancelServiceQoSHistory: ros.slros2.internal.block.SendActionGoalBlockMask.dispatch('qosHistorySelect',gcb,'CancelService');
      mask TypeOptions CancelServiceQoSDepth: SendGoal/CancelServiceQoSDepth
      mask TypeOptions CancelServiceQoSReliability: SendGoal/CancelServiceQoSReliability
      mask TypeOptions CancelServiceQoSDurability: SendGoal/CancelServiceQoSDurability
      mask TypeOptions CancelServiceQoSDeadline: SendGoal/CancelServiceQoSDeadline
      mask TypeOptions CancelServiceQoSLifespan: SendGoal/CancelServiceQoSLifespan
      mask TypeOptions CancelServiceQoSLiveliness: SendGoal/CancelServiceQoSLiveliness
      mask TypeOptions CancelServiceQoSLeaseDuration: SendGoal/CancelServiceQoSLeaseDuration
      mask TypeOptions FeedbackTopicQoSHistory: SendGoal/FeedbackTopicQoSHistory
      mask Callback FeedbackTopicQoSHistory: ros.slros2.internal.block.SendActionGoalBlockMask.dispatch('qosHistorySelect',gcb,'FeedbackTopic');
      mask TypeOptions FeedbackTopicQoSReliability: SendGoal/FeedbackTopicQoSReliability
      mask TypeOptions FeedbackTopicQoSDepth: SendGoal/FeedbackTopicQoSDepth
      mask TypeOptions FeedbackTopicQoSDurability: SendGoal/FeedbackTopicQoSDurability
      mask TypeOptions FeedbackTopicQoSDeadline: SendGoal/FeedbackTopicQoSDeadline
      mask TypeOptions FeedbackTopicQoSLifespan: SendGoal/FeedbackTopicQoSLifespan
      mask TypeOptions FeedbackTopicQoSLiveliness: SendGoal/FeedbackTopicQoSLiveliness
      mask TypeOptions FeedbackTopicQoSLeaseDuration: SendGoal/FeedbackTopicQoSLeaseDuration
      mask TypeOptions StatusTopicQoSHistory: SendGoal/StatusTopicQoSHistory
      mask Callback StatusTopicQoSHistory: ros.slros2.internal.block.SendActionGoalBlockMask.dispatch('qosHistorySelect',gcb,'StatusTopic');
      mask TypeOptions StatusTopicQoSDepth: SendGoal/StatusTopicQoSDepth
      mask TypeOptions StatusTopicQoSReliability: SendGoal/StatusTopicQoSReliability
      mask TypeOptions StatusTopicQoSDurability: SendGoal/StatusTopicQoSDurability
      mask TypeOptions StatusTopicQoSDeadline: SendGoal/StatusTopicQoSDeadline
      mask TypeOptions StatusTopicQoSLifespan: SendGoal/StatusTopicQoSLifespan
      mask TypeOptions StatusTopicQoSLiveliness: SendGoal/StatusTopicQoSLiveliness
      mask TypeOptions StatusTopicQoSLeaseDuration: SendGoal/StatusTopicQoSLeaseDuration
      mask DialogControl id_netAddrLink Prompt: ros:slros2:blockmask:ConfigNetworkAddrLinkText
      mask DialogControl id_netAddrLink Callback: ros.slros2.internal.block.SubscribeBlockMask.dispatch('configureNetworkAddrDlg',gcb);
      mask DialogControl Container3 Prompt: ros:slros2:blockmask:PubSubMainTab
      mask DialogControl actionSource Prompt: Source:
      mask DialogControl action Prompt: Name:
      mask DialogControl id_actionSelectBtn Prompt: ros:slros2:blockmask:SelectPrompt
      mask DialogControl id_actionSelectBtn Callback: ros.slros2.internal.block.SendActionGoalBlockMask.dispatch('actionSelect',gcb,'ros.slros2.internal.dlg.ActionSelector');
      mask DialogControl actionType Prompt: Type:
      mask DialogControl id_actTypeSelectBtn Prompt: ros:slros2:blockmask:SelectPrompt
      mask DialogControl id_actTypeSelectBtn Callback: ros.slros2.internal.block.SendActionGoalBlockMask.dispatch('actionTypeSelect',gcb,'ros.slros2.internal.dlg.ActionTypeSelector');
      mask DialogControl PairedBlkText Prompt: ros:slros2:blockmask:PairedMonitorGoalBlkPrompt
      mask DialogControl PairedBlkLink Prompt: ros2lib/Monitor Action Goal
      mask DialogControl PairedBlkLink Callback: ros.slros.internal.ROSUtil.addMonitorAndSendActionGoalBlockPair(bdroot,'ros2lib/Monitor Action Goal',gcb)
      mask DialogControl ShowErrorCodeOutput Prompt: Show ErrorCode output port
      mask DialogControl Container4 Prompt: ros:slros2:blockmask:PubSubQOSTab
      mask DialogControl Container5 Prompt: ros:slros2:blockmask:GoalServiceQoSPrompt
      mask DialogControl GoalServiceQoSHistory Prompt: History:
      mask DialogControl GoalServiceQoSDepth Prompt: Depth:
      mask DialogControl GoalServiceQoSReliability Prompt: Reliability:
      mask DialogControl GoalServiceQoSDurability Prompt: Durability:
      mask DialogControl GoalServiceQoSDeadline Prompt: Deadline:
      mask DialogControl GoalServiceQoSLifespan Prompt: Lifespan:
      mask DialogControl GoalServiceQoSLiveliness Prompt: Liveliness:
      mask DialogControl GoalServiceQoSLeaseDuration Prompt: Lease Duration:
      mask DialogControl Container6 Prompt: ros:slros2:blockmask:ResultServiceQoSPrompt
      mask DialogControl ResultServiceQoSHistory Prompt: History:
      mask DialogControl ResultServiceQoSDepth Prompt: Depth:
      mask DialogControl ResultServiceQoSReliability Prompt: Reliability:
      mask DialogControl ResultServiceQoSDurability Prompt: Durability:
      mask DialogControl ResultServiceQoSDeadline Prompt: Deadline:
      mask DialogControl ResultServiceQoSLifespan Prompt: Lifespan:
      mask DialogControl ResultServiceQoSLiveliness Prompt: Liveliness:
      mask DialogControl ResultServiceQoSLeaseDuration Prompt: Lease Duration:
      mask DialogControl Container7 Prompt: ros:slros2:blockmask:CancelServiceQoSPrompt
      mask DialogControl CancelServiceQoSHistory Prompt: History:
      mask DialogControl CancelServiceQoSDepth Prompt: Depth:
      mask DialogControl CancelServiceQoSReliability Prompt: Reliability:
      mask DialogControl CancelServiceQoSDurability Prompt: Durability:
      mask DialogControl CancelServiceQoSDeadline Prompt: Deadline:
      mask DialogControl CancelServiceQoSLifespan Prompt: Lifespan:
      mask DialogControl CancelServiceQoSLiveliness Prompt: Liveliness:
      mask DialogControl CancelServiceQoSLeaseDuration Prompt: Lease Duration:
      mask DialogControl Container8 Prompt: ros:slros2:blockmask:FeedbackTopicQoSPrompt
      mask DialogControl FeedbackTopicQoSHistory Prompt: History:
      mask DialogControl FeedbackTopicQoSReliability Prompt: Reliability:
      mask DialogControl FeedbackTopicQoSDepth Prompt: Depth:
      mask DialogControl FeedbackTopicQoSDurability Prompt: Durability:
      mask DialogControl FeedbackTopicQoSDeadline Prompt: Deadline:
      mask DialogControl FeedbackTopicQoSLifespan Prompt: Lifespan:
      mask DialogControl FeedbackTopicQoSLiveliness Prompt: Liveliness:
      mask DialogControl FeedbackTopicQoSLeaseDuration Prompt: Lease Duration:
      mask DialogControl Container9 Prompt: ros:slros2:blockmask:StatusTopicQoSPrompt
      mask DialogControl StatusTopicQoSHistory Prompt: History:
      mask DialogControl StatusTopicQoSDepth Prompt: Depth:
      mask DialogControl StatusTopicQoSReliability Prompt: Reliability:
      mask DialogControl StatusTopicQoSDurability Prompt: Durability:
      mask DialogControl StatusTopicQoSDeadline Prompt: Deadline:
      mask DialogControl StatusTopicQoSLifespan Prompt: Lifespan:
      mask DialogControl StatusTopicQoSLiveliness Prompt: Liveliness:
      mask DialogControl StatusTopicQoSLeaseDuration Prompt: Lease Duration:
      mask Display:
      | color('black');
      | text(0.5, 0.15, '/fibonacci', 'horizontalAlignment', 'center');
      | port_label('input', 1, 'Goal');
      | port_label('input', 2, 'Enable');
      | port_label('output', 1, 'UUID');
      | port_label('output', 2, 'ErrorCode');
  Send Service Response : Subsystem  InitFcn=|  mask(ROS2 Send Service Response){service=/my_service, serviceType=std_srvs/Empty, BlockId=ServRec_ros2lib_224}
      | ros.slros.internal.block.errorIfBlocksConflict(bdroot(gcb));
      | ros.slros.internal.ROSUtil.checkSvcServerBlkAvailability(gcb);
      mask prompts: service "ros:slros:svccaller:NamePrompt"; serviceType "ros:slros:svccaller:TypePrompt"; BlockId "Simulink Block Identifier:"
      mask help: ros:slros2:blockmask:SendResponseDescription
      mask init:
      | ros.slros2.internal.block.SendResponseBlockMask.dispatch('maskInitialize', gcb);
      settings: CopyFcn=ros.slros2.internal.block.SendResponseBlockMask.dispatch('copyBlockInit',gcb);  DeleteFcn=ros.slros.internal.ROSUtil.removeBlkPairingRegistration(gcb);
      mask Help: eval('ros.slros.internal.helpview("ros2SendResponseBlock")');
      mask TypeOptions service: SvcSenderObj/ServiceName
      mask Callback service: ros.slros2.internal.block.SendResponseBlockMask.dispatch('updateSubsystem', gcb);
      mask TypeOptions serviceType: SvcSenderObj/ServiceType
      mask Callback serviceType: ros.slros2.internal.block.SendResponseBlockMask.dispatch('updateSubsystem', gcb);
      mask TypeOptions BlockId: SvcSenderObj/BlockId
      mask DialogControl service Prompt: Name:
      mask DialogControl serviceType Prompt: Type:
      mask DialogControl PairedBlkText Prompt: ros:slros2:blockmask:PairedReceiveBlkPrompt
      mask DialogControl PairedBlkLink Prompt: ros2lib/Receive Service Request
      mask DialogControl PairedBlkLink Callback: ros.slros.internal.ROSUtil.addServerResponseBlockPair(bdroot, 'ros2lib/Receive Service Request', gcb);
      mask Display:
      | color('black');
      | text(0.5, 0.15, '/my_service', 'horizontalAlignment', 'center');
      | port_label('input', 1, 'Resp');
  Subscribe : Subsystem  LoadFcn=ros.slros2.internal.block.SubscribeBlockMask.messageLoadFcn(gcb);  InitFcn=ros.slros.internal.block.errorIfBlocksConflict(bdroot(gcb));  mask(ROS2 Subscribe){topicSource=Select from ROS network, topic=/my_topic, messageType=geometry_msgs/Point, sampleTime=-1, QOSHistory=Keep last, QOSDepth=10, QOSReliability=Reliable, QOSDurability=Volatile, QOSDeadline=Inf, QOSLifespan=Inf, QOSLiveliness=Automatic, QOSLeaseDuration=Inf, QOSAvoidROSNamespaceConventions=off}
      mask prompts: topicSource "ros:slros:blockmask:TopicSourcePrompt"; topic "ros:slros:blockmask:TopicPrompt"; messageType "ros:slros:blockmask:MessageTypePrompt"; sampleTime "ros:slros:blockmask:SampleTimePrompt"; QOSHistory "ros:slros2:blockmask:QOSHistoryPrompt"; QOSDepth "ros:slros2:blockmask:QOSDepthPrompt"; QOSReliability "ros:slros2:blockmask:QOSReliabilityPrompt"; QOSDurability "ros:slros2:blockmask:QOSDurabilityPrompt"; QOSDeadline "ros:slros2:blockmask:QOSDeadlinePrompt"; QOSLifespan "ros:slros2:blockmask:QOSLifespanPrompt"; QOSLiveliness "ros:slros2:blockmask:QOSLivelinessPrompt"; QOSLeaseDuration "ros:slros2:blockmask:QOSLeaseDurationPrompt"; QOSAvoidROSNamespaceConventions "ros:slros2:blockmask:QOSAvoidROSNamespaceConventionsPrompt"
      mask help: ros:slros:blockmask:SubscriberDescription
      mask init:
      | ros.slros2.internal.block.SubscribeBlockMask.dispatch('maskInitialize', gcb);
      settings: ModelCloseFcn=ros.slros2.internal.bus.Util.clearSLBusesInGlobalScope(gcb);
      mask Help: eval('ros.slros.internal.helpview(''ros2SubscribeBlock'')');
      mask TypeOptions topicSource: ros:slros2:blockmask:TopicSourceFromNetwork | ros:slros2:blockmask:TopicSourceSpecifyOwn
      mask Callback topicSource: ros.slros2.internal.block.SubscribeBlockMask.dispatch('topicSourceSelect', gcb);
      mask Callback topic: ros.slros2.internal.block.SubscribeBlockMask.dispatch('topicEdit', gcb);
      mask Callback messageType: ros.slros2.internal.block.SubscribeBlockMask.dispatch('messageTypeEdit', gcb);
      mask TypeOptions sampleTime: Constant/SampleTime
      mask TypeOptions QOSHistory: SourceBlock/QOSHistory
      mask Callback QOSHistory: ros.slros2.internal.block.QOSSettingsMask.qosHistorySelect(gcb);
      mask TypeOptions QOSDepth: SourceBlock/QOSDepth
      mask TypeOptions QOSReliability: SourceBlock/QOSReliability
      mask TypeOptions QOSDurability: SourceBlock/QOSDurability
      mask TypeOptions QOSDeadline: SourceBlock/QOSDeadline
      mask TypeOptions QOSLifespan: SourceBlock/QOSLifespan
      mask TypeOptions QOSLiveliness: SourceBlock/QOSLiveliness
      mask TypeOptions QOSLeaseDuration: SourceBlock/QOSLeaseDuration
      mask TypeOptions QOSAvoidROSNamespaceConventions: SourceBlock/QOSAvoidROSNamespaceConventions
      mask DialogControl id_netAddrLink Prompt: ros:slros2:blockmask:ConfigNetworkAddrLinkText
      mask DialogControl id_netAddrLink Callback: ros.slros2.internal.block.SubscribeBlockMask.dispatch('configureNetworkAddrDlg', gcb);
      mask DialogControl Container13 Prompt: ros:slros2:blockmask:PubSubMainTab
      mask DialogControl topicSource Prompt: Topic source:
      mask DialogControl topic Prompt: Topic:
      mask DialogControl id_topicSelectBtn Prompt: ros:slros:blockmask:SelectPrompt
      mask DialogControl id_topicSelectBtn Callback: ros.slros2.internal.block.SubscribeBlockMask.dispatch('topicSelect', gcb, 'ros.slros2.internal.dlg.TopicSelector');
      mask DialogControl messageType Prompt: Message type:
      mask DialogControl id_msgTypeSelectBtn Prompt: ros:slros:blockmask:SelectPrompt
      mask DialogControl id_msgTypeSelectBtn Callback: ros.slros2.internal.block.SubscribeBlockMask.dispatch('messageTypeSelect', gcb, 'ros.slros2.internal.dlg.MessageTypeSelector');
      mask DialogControl sampleTime Prompt: Sample time:
      mask DialogControl id_cgContainer Prompt: ros:slros2:blockmask:PubSubQOSTab
      mask DialogControl QOSHistory Prompt: History:
      mask DialogControl QOSDepth Prompt: Depth:
      mask DialogControl QOSReliability Prompt: Reliability:
      mask DialogControl QOSDurability Prompt: Durability:
      mask DialogControl QOSDeadline Prompt: Deadline:
      mask DialogControl QOSLifespan Prompt: Lifespan:
      mask DialogControl QOSLiveliness Prompt: Liveliness:
      mask DialogControl QOSLeaseDuration Prompt: Lease Duration:
      mask DialogControl QOSAvoidROSNamespaceConventions Prompt: Avoid ROS Namespace Conventions
      mask Display:
      | color('black');
      | text(0.45, 0.15, '/my_topic', 'horizontalAlignment', 'center');
      | port_label('output', 1, 'IsNew');
      | port_label('output', 2, 'Msg');
  Write Image : Subsystem  InitFcn=|  mask(ROS2 Write Image){ImageEncoding=rgb8, EncodingStruct=ros.msg.sensor_msgs.internal.ImageEncoding.info(coder.const('rgb8')), HasAlpha=off, messageType=sensor_msgs/Image}
      | ros.slros.internal.block.errorIfBlocksConflict(bdroot(gcb));
      | ros.slros2.internal.block.WriteImageBlockMask.dispatch('maskInitialize', gcb);
      mask prompts: ImageEncoding "ros:slros2:blockmask:ImageEncodingPrompt"
      mask init:
      | ros.slros2.internal.block.WriteImageBlockMask.dispatch('maskInitialize', gcb);
      mask Help: eval('ros.slros.internal.helpview(''ros2WriteImBlock'')');
      mask TypeOptions ImageEncoding: rgb8 | rgba8 | rgb16 | rgba16 | bgr8 | bgra8 | bgr16 | bgra16 | mono8 | mono16 | 32fc1 | 32fc2 | 32fc3 | 32fc4 | 64fc1 | 64fc2 | 64fc3 | 64fc4 | 8uc1 | 8uc2 | 8uc3 | 8uc4 | 8sc1 | 8sc2 | 8sc3 | 8sc4 | 16uc1 | 16uc2 | 16uc3 | 16uc4 | 16sc1 | 16sc2 | 16sc3 | 16sc4 | 32sc1 | 32sc2 | 32sc3 | 32sc4
      mask DialogControl DescGroupVar Prompt: ros:slros2:blockmask:WriteImageTitle
      mask DialogControl DescTextVar Prompt: ros:slros2:blockmask:WriteImageDescription
      mask DialogControl Settings Prompt: ros:slros2:blockmask:ImagePropertiesPrompt
      mask DialogControl ImageEncoding Prompt: Image encoding:
      mask Display: port_label('input',1,'Image');port_label('output',1,'Msg');
  Write Point Cloud : Subsystem  InitFcn=|  mask(ROS2 Write Point Cloud){messageType=sensor_msgs/PointCloud2, Encoding=none, HasRGB=false, HasAlpha=false, HasIntensityCheck=off, HasIntensity=false, FieldNamesStruct=struct('x', 'single', 'y', 'single', 'z', 'single')}
      | ros.slros.internal.block.errorIfBlocksConflict(bdroot(gcb));
      | ros.slros2.internal.block.WritePointCloudBlockMask.dispatch('maskInitialize', gcb);
      mask prompts: Encoding "ros:slros2:blockmask:SelectRGBInputPrompt"; HasIntensityCheck "ros:slros2:blockmask:WriteIntensityFieldPrompt"
      mask init:
      | ros.slros2.internal.block.WritePointCloudBlockMask.dispatch('maskInitialize', gcb);
      mask Help: eval('ros.slros.internal.helpview(''ros2WritePCBlock'')');
      mask TypeOptions Encoding: none | rgb | rgba
      mask DialogControl DescGroupVar Prompt: ros:slros2:blockmask:WritePointCloudTitle
      mask DialogControl DescTextVar Prompt: ros:slros2:blockmask:WritePointCloudDescription
      mask DialogControl ParameterGroupVar Prompt: ros:slros2:blockmask:InputConfiguration
      mask DialogControl Encoding Prompt: Select color field
      mask DialogControl HasIntensityCheck Prompt: Write to Intensity field
      mask Display: port_label('input', 1, 'XYZ'); port_label('output', 1, 'Msg');
